simulink model "zouzhihua_2016a"  (R2018b)
settings: Solver=ode4  StartTime=0.0  StopTime=15  FixedStep=0.001  RelTol=1e-3  EnableMultiTasking=on
settings Model: ExtModeTrigMode=oneshot  ExtModeArmWhenConnect=off  Creator=hp  LastModifiedBy=Administrator
settings SolverCC: AlgebraicLoopSolver=LineSearch
settings DataIOCC: SaveFormat=Array  SignalLoggingSaveFormat=ModelDataLogs  SignalLoggingName=sigsOut
settings OptimizationCC: BooleanDataType=off  ExpressionDepthLimit=2147483647  InitFltsAndDblsToZero=on  LifeSpan=inf
settings DebuggingCC: SaveWithParameterizedLinksMsg=none  UnderspecifiedInitializationDetection=Classic  MergeDetectMultiDrivingBlocksExec=none  SignalResolutionControl=TryResolveAllWithWarning  MultiTaskDSMMsg=warning  MultiTaskCondExecSysMsg=none  FcnCallInpInsideContextMsg=warning  StateNameClashWarn=warning  SFUnexpectedBacktrackingDiag=warning  SFNoUnconditionalDefaultTransitionDiag=warning
settings HardwareCC: ProdBitPerPointer=32  ProdBitPerSizeT=32  ProdBitPerPtrDiffT=32  ProdLargestAtomicFloat=None  ProdIntDivRoundTo=Undefined  ProdEndianess=Unspecified  ProdWordSize=32  ProdHWDeviceType=32-bit Generic  TargetUnknown=on
settings ModelReferenceCC: PropagateSignalLabelsOutOfModel=off
settings SFSimCC: SimUseLocalCustomCode=off
settings RTWCC: RTWUseLocalCustomCode=off
settings CodeAppCC: StateflowObjectComments=on
settings GRTTargetCC: TargetFcnLib=ansi_tfl_tmw.mat  TargetLangStandard=C89/C90 (ANSI)  CombineOutputUpdateFcns=off  GRTInterface=on
settings ConfigComp: CovMetricSettings=dw  CovHtmlReporting=on  CovSaveCumulativeToWorkspaceVar=on  CovSaveSingleToWorkspaceVar=on  CovExternalEMLEnable=off

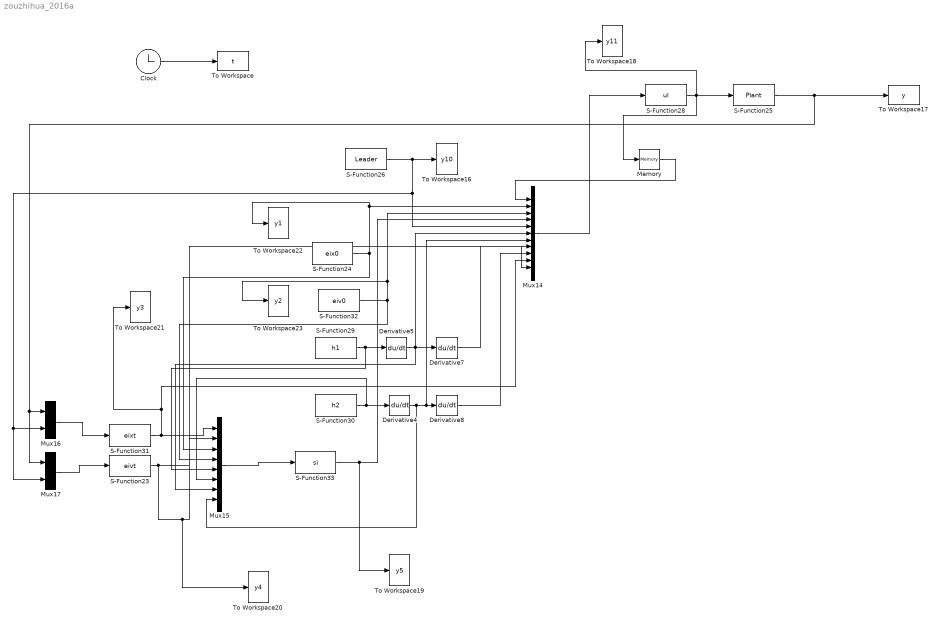
== system zouzhihua_2016a ==
  Clock : Clock
  Derivative{4..5,7..8} (4 alike) : Derivative
  Memory : Memory
  Mux14 : Mux  Inputs=11
  Mux15 : Mux  Inputs=8
  Mux16 : Mux  Inputs=2
  Mux17 : Mux  Inputs=2
  S-Function23 : S-Function  FunctionName=eivt  SFunctionDeploymentMode=off  EnableBusSupport=off
  S-Function24 : S-Function  FunctionName=eix0  SFunctionDeploymentMode=off  EnableBusSupport=off
  S-Function25 : S-Function  FunctionName=Plant  SFunctionDeploymentMode=off  EnableBusSupport=off
  S-Function26 : S-Function  FunctionName=Leader  SFunctionDeploymentMode=off  EnableBusSupport=off
  S-Function28 : S-Function  FunctionName=ul  SFunctionDeploymentMode=off  EnableBusSupport=off
  S-Function29 : S-Function  FunctionName=h1  SFunctionDeploymentMode=off  EnableBusSupport=off
  S-Function30 : S-Function  FunctionName=h2  SFunctionDeploymentMode=off  EnableBusSupport=off
  S-Function31 : S-Function  FunctionName=eixt  SFunctionDeploymentMode=off  EnableBusSupport=off
  S-Function32 : S-Function  FunctionName=eiv0  SFunctionDeploymentMode=off  EnableBusSupport=off
  S-Function33 : S-Function  FunctionName=si  SFunctionDeploymentMode=off  EnableBusSupport=off
  To Workspace : ToWorkspace  VariableName=t  SampleTime=-1
  To Workspace16 : ToWorkspace  VariableName=y10  SampleTime=-1
  To Workspace17 : ToWorkspace  VariableName=y  SampleTime=-1
  To Workspace18 : ToWorkspace  VariableName=y11  SampleTime=-1
  To Workspace19 : ToWorkspace  VariableName=y5  SampleTime=-1
  To Workspace20 : ToWorkspace  VariableName=y4  SampleTime=-1
  To Workspace21 : ToWorkspace  VariableName=y3  SampleTime=-1
  To Workspace22 : ToWorkspace  VariableName=y1  SampleTime=-1
  To Workspace23 : ToWorkspace  VariableName=y2  SampleTime=-1
  wires:
  Clock/1 -> To Workspace/1
  S-Function26/1 -> Mux17/2, Mux16/2, Mux14/5, To Workspace16/1
  Mux14/1 -> S-Function28/1
  S-Function28/1 -> Memory/1, To Workspace18/1, S-Function25/1
  S-Function29/1 -> Mux15/5, Derivative5/1
  S-Function30/1 -> Mux15/6, Derivative4/1
  Derivative5/1 -> Mux14/6, Mux15/7, Derivative7/1
  S-Function24/1 -> Mux15/3, To Workspace22/1, Mux14/2
  S-Function32/1 -> Mux15/4, To Workspace23/1, Mux14/3
  Derivative4/1 -> Mux15/8, Mux14/7, Derivative8/1
  S-Function31/1 -> To Workspace21/1, Mux14/10, Mux15/1
  S-Function23/1 -> To Workspace20/1, Mux14/11, Mux15/2
  Mux15/1 -> S-Function33/1
  S-Function25/1 -> Mux17/1, Mux16/1, To Workspace17/1
  S-Function33/1 -> To Workspace19/1, Mux14/4
  Derivative7/1 -> Mux14/8
  Derivative8/1 -> Mux14/9
  Mux17/1 -> S-Function23/1
  Mux16/1 -> S-Function31/1
  Memory/1 -> Mux14/1
